simulink subsystem "PvtSubSys_VSM_LngHMI"  (R2020b)
settings: Solver=VariableStepAuto  StartTime=0.0  StopTime=10.0  RelTol=1e-3
undefined symbols (not defined in the file): ACC_STATE, HWA_STATE, P_VSM_HMI_Curve, P_VSM_HMI_CurveTime, P_VSM_LSMC_SampleTime, TJA_STATE
libraries: simulink x101
settings Model: Creator=GW00133806  LastModifiedBy=GW00201299

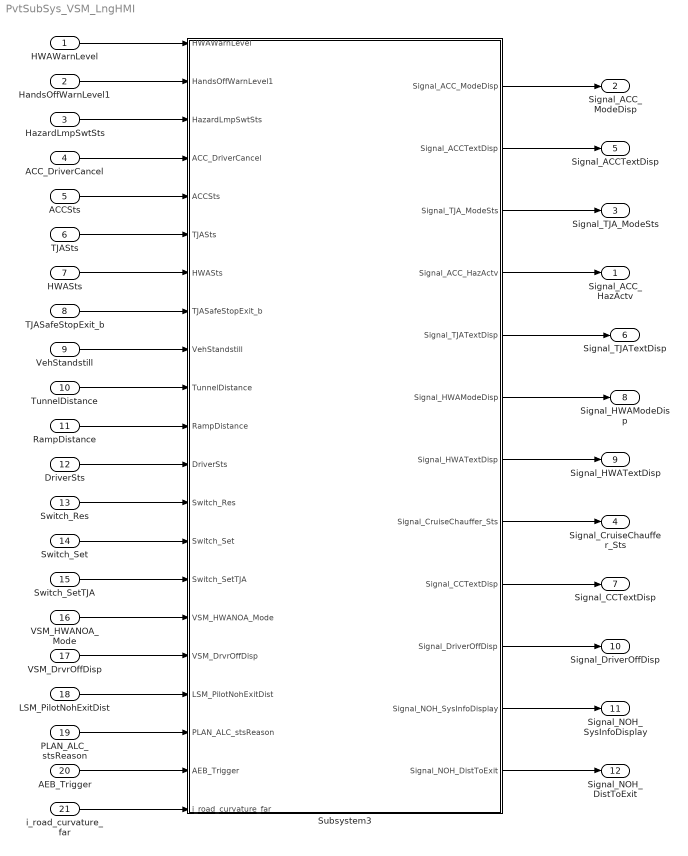
== system PvtSubSys_VSM_LngHMI ==
  HWAWarnLevel : Inport  OutDataTypeStr=uint8
  HandsOffWarnLevel1 : Inport  Port=2  OutDataTypeStr=uint8
  HazardLmpSwtSts : Inport  Port=3  OutDataTypeStr=boolean
  ACC_DriverCancel : Inport  Port=4  OutDataTypeStr=boolean
  ACCSts : Inport  Port=5  OutDataTypeStr=Enum: ACC_STATE
  TJASts : Inport  Port=6  OutDataTypeStr=Enum: TJA_STATE
  HWASts : Inport  Port=7  OutDataTypeStr=Enum: HWA_STATE
  TJASafeStopExit_b : Inport  Port=8  OutDataTypeStr=boolean
  VehStandstill : Inport  Port=9  OutDataTypeStr=uint8
  TunnelDistance : Inport  Port=10  OutDataTypeStr=uint16
  RampDistance : Inport  Port=11  OutDataTypeStr=uint16
  DriverSts : Inport  Port=12  OutDataTypeStr=uint8
  Switch_Res : Inport  Port=13  OutDataTypeStr=boolean
  Switch_Set : Inport  Port=14  OutDataTypeStr=boolean
  Switch_SetTJA : Inport  Port=15  OutDataTypeStr=boolean
  VSM_HWANOA_Mode : Inport  Port=16
  VSM_DrvrOffDisp : Inport  Port=17
  LSM_PilotNohExitDist : Inport  Port=18
  PLAN_ALC_stsReason : Inport  Port=19
  AEB_Trigger : Inport  Port=20
  i_road_curvature_far : Inport  Port=21
  Subsystem3 : Subsystem
  Signal_ACC_HazActv : Outport  OutDataTypeStr=uint8
  Signal_ACC_ModeDisp : Outport  Port=2  OutDataTypeStr=uint8
  Signal_TJA_ModeSts : Outport  Port=3  OutDataTypeStr=uint8
  Signal_CruiseChauffer_Sts : Outport  Port=4
  Signal_ACCTextDisp : Outport  Port=5  OutDataTypeStr=uint8
  Signal_TJATextDisp : Outport  Port=6  OutDataTypeStr=uint8
  Signal_CCTextDisp : Outport  Port=7
  Signal_HWAModeDisp : Outport  Port=8  OutDataTypeStr=uint8
  Signal_HWATextDisp : Outport  Port=9  OutDataTypeStr=uint8
  Signal_DriverOffDisp : Outport  Port=10
  Signal_NOH_SysInfoDisplay : Outport  Port=11
  Signal_NOH_DistToExit : Outport  Port=12
  wires:
  i_road_curvature_far/1 -> Subsystem3/21(i_road_curvature_far)
  AEB_Trigger/1 -> Subsystem3/20(AEB_Trigger)
  VSM_DrvrOffDisp/1 -> Subsystem3/17(VSM_DrvrOffDisp)
  VSM_HWANOA_Mode/1 -> Subsystem3/16(VSM_HWANOA_Mode)
  Switch_Set/1 -> Subsystem3/14(Switch_Set)
  TJASts/1 -> Subsystem3/6(TJASts)
  ACCSts/1 -> Subsystem3/5(ACCSts)
  HandsOffWarnLevel1/1 -> Subsystem3/2(HandsOffWarnLevel1)
  VehStandstill/1 -> Subsystem3/9(VehStandstill)
  ACC_DriverCancel/1 -> Subsystem3/4(ACC_DriverCancel)
  TJASafeStopExit_b/1 -> Subsystem3/8(TJASafeStopExit_b)
  TunnelDistance/1 -> Subsystem3/10(TunnelDistance)
  Switch_Res/1 -> Subsystem3/13(Switch_Res)
  RampDistance/1 -> Subsystem3/11(RampDistance)
  HWASts/1 -> Subsystem3/7(HWASts)
  HazardLmpSwtSts/1 -> Subsystem3/3(HazardLmpSwtSts)
  Subsystem3/7(Signal_HWATextDisp) -> Signal_HWATextDisp/1
  Subsystem3/1(Signal_ACC_ModeDisp) -> Signal_ACC_ModeDisp/1
  Subsystem3/8(Signal_CruiseChauffer_Sts) -> Signal_CruiseChauffer_Sts/1
  Subsystem3/9(Signal_CCTextDisp) -> Signal_CCTextDisp/1
  Switch_SetTJA/1 -> Subsystem3/15(Switch_SetTJA)
  Subsystem3/3(Signal_TJA_ModeSts) -> Signal_TJA_ModeSts/1
  Subsystem3/4(Signal_ACC_HazActv) -> Signal_ACC_HazActv/1
  HWAWarnLevel/1 -> Subsystem3/1(HWAWarnLevel)
  Subsystem3/2(Signal_ACCTextDisp) -> Signal_ACCTextDisp/1
  DriverSts/1 -> Subsystem3/12(DriverSts)
  Subsystem3/5(Signal_TJATextDisp) -> Signal_TJATextDisp/1
  Subsystem3/6(Signal_HWAModeDisp) -> Signal_HWAModeDisp/1
  Subsystem3/10(Signal_DriverOffDisp) -> Signal_DriverOffDisp/1
  LSM_PilotNohExitDist/1 -> Subsystem3/18(LSM_PilotNohExitDist)
  Subsystem3/11(Signal_NOH_SysInfoDisplay) -> Signal_NOH_SysInfoDisplay/1
  Subsystem3/12(Signal_NOH_DistToExit) -> Signal_NOH_DistToExit/1
  PLAN_ALC_stsReason/1 -> Subsystem3/19(PLAN_ALC_stsReason)

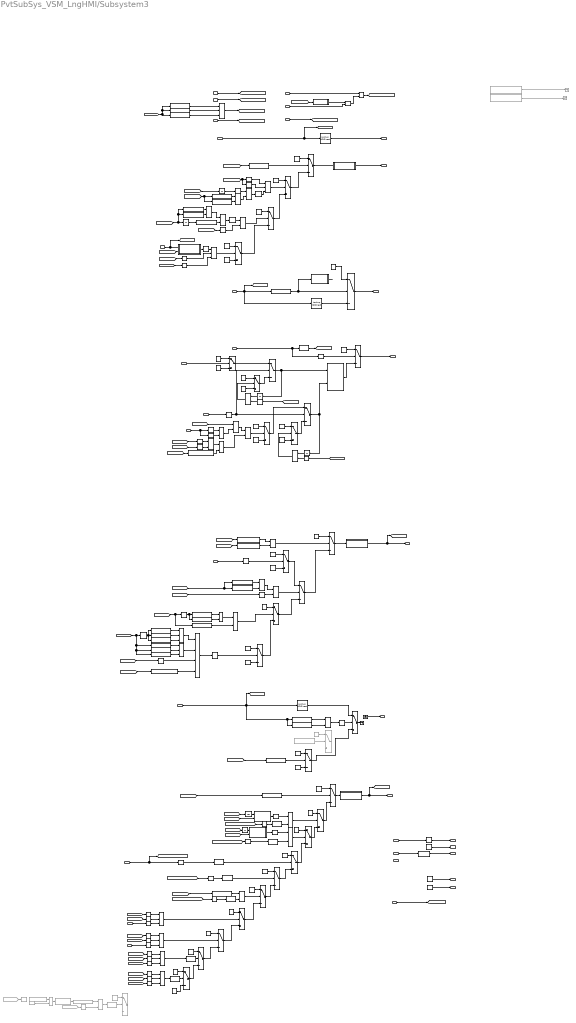
== system PvtSubSys_VSM_LngHMI/Subsystem3 ==
  note: 优先报ACC故障
  note: 0x0:No display
      | 0x1:Unable to activate TJA/ICA due to other limitation
      | 0x2:TJA/ICA active control is cancelled
      | 0x3:TJA/ICA   temporarily unavailable
      | 0x4:Current IGN Cycle Function Inhibit
      | 0x5：TJA Active
      | 0x6-0x7:Resvered
  note: 0x0:OFF
      | 0x1:Safstop
      | 0x2:Passive
      | 0x3:Ready
      | 0x4:Active
      | 0x5:Override
      | 0x6:Slow retreat
      | 0x7:Standstill
      | 0x8-0xE:Reserved
      | 0xF:Fault
  note: 0x0:No display
      | 0x1:Unable to activate HWA due to other limitation
      | 0x2:HWA active control is cancelled
      | 0x3:Turn off the turn light
      | 0x4:Active confirm
      | 0x5:Overtime for lane change
      | 0x6:lane change is cancelled
      | 0x7:HWA temporary unavailable
      | 0x8:Speed is too low to support lane change
      | 0x9:HWA need to restart the engine
      | 0xA:Take over request
      | 0xB: Please Keep Attention
      | 0xC:To cross the tunnel, please take over  in time
      | 0xD:Have a branch road ahead. Please take over in time
      | 0xE-0xF:Reserve
  note: 0x0:OFF mode
      | 0x1:Passive mode
      | 0x2:Active mode
      | 0x3:Ready
      | 0x4: Failure
      | 0x5:TJA_Wait状态灯闪闪烁，未确定此效果是否作出
  note: 0x00:No display
      | 0x01:Unable to activate ACC due to speed not achive
      | 0x02:ACC active control is cancelled
      | 0x03:Resvered
      | 0x04:ACC and PEBS temporary unavailable
      | 0x05:Unable to activate ACC due to other limitation(except speed not achive)
      | 0x06:ACC and PEBS error
      | 0x07:ACC temporary unavailable
      | 0x08:ACC Active
      | 0x09:Blindness
      | 0x0A-0x1F:Resvered
  note: 0x00:OFF Mode
      | 0x01:Passive Mode
      | 0x02:StandBy Mode
      | 0x03:Active-Control Mode
      | 0x04:Brake-Only Mode
      | 0x05:Override
      | 0X06:Reserved
      | 0X07:ACC and PEBS Failure mode
      | 0x08:ACC Failure mode
      | 0x09-0x1F:Reserved
  note: 2020.12.15
      | 1、新架构更新，初版
      |
      | 2020.12.29
      | 1、临时增加VSM_DrvrOffDisp信号输出到CCTextDisp上给HMI；
      | 2、修改HWA文字提醒输出3和5和8的逻辑；
      | 3、ACC仪表显示状态延迟2周期，以修改TJA激活时先报ACC激活的问题；
      | 4、TJA_Wait输出active到仪表；
      | 2021.1.5
      | 1、修改换道取消的发送逻辑，及其和换道成功的优先级顺序；
      | 2021.1.19
      | 把HWA的低速提醒限值改为PLAN的标定量；
      | 2021.1.27
      | ACC/TJA激活提醒策略添加；
      | 2021.1.30
      | TJA显示修改；
      | 2021.2.5
      | TJA显示修改；
      | ACC/TJA/HWA取消HMI逻辑修改
      | 2021.2.8
      | ACC/TJA故障显示优先级修改；
      | 2021.2.22
      | 增加NOH相关信号，增加ACCDrvrOffDisp信号；
      | 2021.3.5
      | VSM_HWA_ModeDisp删除override状态
      | 2021.3.12
      | TJA在ACCStandwait时不报退出提醒；
  note: 架构需求车速过低过
      | 高不能换道仅报警一次
  HWAWarnLevel : Inport  OutDataTypeStr=uint8
  HandsOffWarnLevel1 : Inport  Port=2  OutDataTypeStr=uint8
  HazardLmpSwtSts : Inport  Port=3  OutDataTypeStr=boolean
  ACC_DriverCancel : Inport  Port=4  OutDataTypeStr=boolean
  ACCSts : Inport  Port=5  OutDataTypeStr=Enum: ACC_STATE
  TJASts : Inport  Port=6  OutDataTypeStr=Enum: TJA_STATE
  HWASts : Inport  Port=7  OutDataTypeStr=Enum: HWA_STATE
  TJASafeStopExit_b : Inport  Port=8  OutDataTypeStr=boolean
  VehStandstill : Inport  Port=9  OutDataTypeStr=uint8
  TunnelDistance : Inport  Port=10  OutDataTypeStr=uint16
  RampDistance : Inport  Port=11  OutDataTypeStr=uint16
  DriverSts : Inport  Port=12  OutDataTypeStr=uint8
  Switch_Res : Inport  Port=13  OutDataTypeStr=boolean
  Switch_Set : Inport  Port=14  OutDataTypeStr=boolean
  Switch_SetTJA : Inport  Port=15  OutDataTypeStr=boolean
  VSM_HWANOA_Mode : Inport  Port=16
  VSM_DrvrOffDisp : Inport  Port=17
  LSM_PilotNohExitDist : Inport  Port=18
  PLAN_ALC_stsReason : Inport  Port=19
  AEB_Trigger : Inport  Port=20
  i_road_curvature_far : Inport  Port=21
  3-1跳变 : Stateflow chart  TreatAsAtomicUnit=on
  AND : Logic  AllPortsSameDT=off  OutDataTypeStr=boolean
  Abs : Abs  Commented=on
  Chart2 : Stateflow chart  TreatAsAtomicUnit=on
  Chart3 : Stateflow chart  TreatAsAtomicUnit=on
  Compare To Constant1 : simulink/Logic and Bit Operations/Compare To Constant  relop===  const=ACC_STATE.ACC_Failure  OutDataTypeStr=boolean
  Compare To Constant{2,10,12,19,22,40..41,44,47..48,51} (11 alike) : simulink/Logic and Bit Operations/Compare To Constant  relop===  const=1  OutDataTypeStr=boolean
  Compare To Constant104 : simulink/Logic and Bit Operations/Compare To Constant  relop===  const=7  OutDataTypeStr=boolean
  Compare To Constant{27,33,105..106} (4 alike) : simulink/Logic and Bit Operations/Compare To Constant  relop===  const=0  OutDataTypeStr=boolean
  Compare To Constant11 : simulink/Logic and Bit Operations/Compare To Constant  relop===  const=3  OutDataTypeStr=boolean
  Compare To Constant114 : simulink/Logic and Bit Operations/Compare To Constant  Commented=on  relop=>=  const=P_VSM_HMI_Curve  OutDataTypeStr=boolean
  Compare To Constant115 : simulink/Logic and Bit Operations/Compare To Constant  Commented=on  relop=<  const=1  OutDataTypeStr=boolean
  Compare To Constant116 : simulink/Logic and Bit Operations/Compare To Constant  Commented=on  relop=>  const=P_VSM_HMI_CurveTime  OutDataTypeStr=boolean
  Compare To Constant13 : simulink/Logic and Bit Operations/Compare To Constant  Commented=on  relop===  const=1  OutDataTypeStr=boolean
  Compare To Constant14 : simulink/Logic and Bit Operations/Compare To Constant  relop===  const=HWA_STATE.HWA_CCAct  OutDataTypeStr=boolean
  Compare To Constant15 : simulink/Logic and Bit Operations/Compare To Constant  relop===  const=HWA_STATE.HWA_Pause  OutDataTypeStr=boolean
  Compare To Constant16 : simulink/Logic and Bit Operations/Compare To Constant  Commented=on  relop===  const=ACC_STATE.ACC_Override  OutDataTypeStr=boolean
  Compare To Constant17 : simulink/Logic and Bit Operations/Compare To Constant  relop===  const=ACC_STATE.ACC_StandWait  OutDataTypeStr=boolean
  Compare To Constant18 : simulink/Logic and Bit Operations/Compare To Constant  relop=~=  const=ACC_STATE.ACC_StandWait  OutDataTypeStr=boolean
  Compare To Constant20 : simulink/Logic and Bit Operations/Compare To Constant  relop===  const=TJA_STATE.TJA_Idle  OutDataTypeStr=boolean
  Compare To Constant21 : simulink/Logic and Bit Operations/Compare To Constant  relop===  const=2  OutDataTypeStr=boolean
  Compare To Constant23 : simulink/Logic and Bit Operations/Compare To Constant  relop===  const=HWA_STATE.HWA_Error  OutDataTypeStr=boolean
  Compare To Constant24 : simulink/Logic and Bit Operations/Compare To Constant  relop===  const=TJA_STATE.TJA_Idle  OutDataTypeStr=boolean
  Compare To Constant25 : simulink/Logic and Bit Operations/Compare To Constant  relop===  const=TJA_STATE.TJA_SafeStop  OutDataTypeStr=boolean
  Compare To Constant26 : simulink/Logic and Bit Operations/Compare To Constant  relop===  const=TJA_STATE.TJA_Active  OutDataTypeStr=boolean
  Compare To Constant28 : simulink/Logic and Bit Operations/Compare To Constant  relop===  const=TJA_STATE.TJA_Wait  OutDataTypeStr=boolean
  Compare To Constant29 : simulink/Logic and Bit Operations/Compare To Constant  relop===  const=3  OutDataTypeStr=boolean
  Compare To Constant3 : simulink/Logic and Bit Operations/Compare To Constant  relop===  const=ACC_STATE.ACC_Reject  OutDataTypeStr=boolean
  Compare To Constant30 : simulink/Logic and Bit Operations/Compare To Constant  relop===  const=HWA_STATE.HWA_CCAct  OutDataTypeStr=boolean
  Compare To Constant31 : simulink/Logic and Bit Operations/Compare To Constant  relop===  const=TJA_STATE.TJA_Active  OutDataTypeStr=boolean
  Compare To Constant32 : simulink/Logic and Bit Operations/Compare To Constant  relop===  const=TJA_STATE.TJA_Wait  OutDataTypeStr=boolean
  Compare To Constant34 : simulink/Logic and Bit Operations/Compare To Constant  relop===  const=4  OutDataTypeStr=boolean
  Compare To Constant35 : simulink/Logic and Bit Operations/Compare To Constant  relop=~=  const=1  OutDataTypeStr=boolean
  Compare To Constant36 : simulink/Logic and Bit Operations/Compare To Constant  relop=~=  const=4  OutDataTypeStr=boolean
  Compare To Constant37 : simulink/Logic and Bit Operations/Compare To Constant  relop===  const=TJA_STATE.TJA_Ready  OutDataTypeStr=boolean
  Compare To Constant38 : simulink/Logic and Bit Operations/Compare To Constant  relop=~=  const=2  OutDataTypeStr=boolean
  Compare To Constant{39,43,46,49} (4 alike) : simulink/Logic and Bit Operations/Compare To Constant  relop=~=  const=0  OutDataTypeStr=boolean
  Compare To Constant4 : simulink/Logic and Bit Operations/Compare To Constant  relop===  const=ACC_STATE.ACC_Standby  OutDataTypeStr=boolean
  Compare To Constant42 : simulink/Logic and Bit Operations/Compare To Constant  relop=<=  const=300  OutDataTypeStr=boolean
  Compare To Constant45 : simulink/Logic and Bit Operations/Compare To Constant  relop=<=  const=300  OutDataTypeStr=boolean
  Compare To Constant5 : simulink/Logic and Bit Operations/Compare To Constant  relop===  const=2  OutDataTypeStr=boolean
  Compare To Constant50 : simulink/Logic and Bit Operations/Compare To Constant  relop=~=  const=1  OutDataTypeStr=boolean
  Compare To Constant52 : simulink/Logic and Bit Operations/Compare To Constant  relop===  const=TJA_STATE.TJA_SafeStop  OutDataTypeStr=boolean
  Compare To Constant53 : simulink/Logic and Bit Operations/Compare To Constant  relop=~=  const=2  OutDataTypeStr=boolean
  Compare To Constant54 : simulink/Logic and Bit Operations/Compare To Constant  relop===  const=TJA_STATE.TJA_SafeStop  OutDataTypeStr=boolean
  Compare To Constant55 : simulink/Logic and Bit Operations/Compare To Constant  relop===  const=TJA_STATE.TJA_SlowRetreat  OutDataTypeStr=boolean
  Compare To Constant56 : simulink/Logic and Bit Operations/Compare To Constant  relop=~=  const=ACC_STATE.ACC_Failure  OutDataTypeStr=boolean
  Compare To Constant58 : simulink/Logic and Bit Operations/Compare To Constant  relop=~=  const=5  OutDataTypeStr=boolean
  Compare To Constant59 : simulink/Logic and Bit Operations/Compare To Constant  relop===  const=ACC_STATE.ACC_Standby  OutDataTypeStr=boolean
  Compare To Constant6 : simulink/Logic and Bit Operations/Compare To Constant  relop===  const=3  OutDataTypeStr=boolean
  Compare To Constant60 : simulink/Logic and Bit Operations/Compare To Constant  relop===  const=ACC_STATE.ACC_ActiveControl  OutDataTypeStr=boolean
  Compare To Constant61 : simulink/Logic and Bit Operations/Compare To Constant  relop===  const=ACC_STATE.ACC_StandActive  OutDataTypeStr=boolean
  Compare To Constant63 : simulink/Logic and Bit Operations/Compare To Constant  relop===  const=TJA_STATE.TJA_Active  OutDataTypeStr=boolean
  Compare To Constant64 : simulink/Logic and Bit Operations/Compare To Constant  relop===  const=TJA_STATE.TJA_Ready  OutDataTypeStr=boolean
  Compare To Constant65 : simulink/Logic and Bit Operations/Compare To Constant  relop===  const=TJA_STATE.TJA_Error  OutDataTypeStr=boolean
  Compare To Constant66 : simulink/Logic and Bit Operations/Compare To Constant  relop===  const=TJA_STATE.TJA_Wait  OutDataTypeStr=boolean
  Compare To Constant67 : simulink/Logic and Bit Operations/Compare To Constant  relop===  const=TJA_STATE.TJA_Error  OutDataTypeStr=boolean
  Compare To Constant7 : simulink/Logic and Bit Operations/Compare To Constant  relop===  const=4  OutDataTypeStr=boolean
  Compare To Constant8 : simulink/Logic and Bit Operations/Compare To Constant  relop===  const=TJA_STATE.TJA_SlowRetreat  OutDataTypeStr=boolean
  Constant{,4,6..7,15,23,31,35,37,39} (10 alike) : Constant  Value=0  OutDataTypeStr=uint8
  Constant1 : Constant  Value=7  OutDataTypeStr=uint8
  Constant10 : Constant  Value=4  OutDataTypeStr=uint8
  Constant11 : Constant  Value=3  OutDataTypeStr=uint8
  Constant12 : Constant  Value=4  OutDataTypeStr=uint8
  Constant13 : Constant  OutDataTypeStr=uint8
  Constant{3,5,14,29} (4 alike) : Constant  Value=2  OutDataTypeStr=uint8
  Constant16 : Constant  Value=7  OutDataTypeStr=uint8
  Constant17 : Constant  Commented=on  Value=301  OutDataTypeStr=uint16
  Constant18 : Constant  Commented=on  Value=38252005  OutDataTypeStr=uint32
  Constant19 : Constant  Value=3  OutDataTypeStr=uint8
  Constant{2,21,32..33} (4 alike) : Constant  Value=5  OutDataTypeStr=uint8
  Constant22 : Constant  Value=8  OutDataTypeStr=uint8
  Constant24 : Constant  Value=12  OutDataTypeStr=uint8
  Constant25 : Constant  Value=13  OutDataTypeStr=uint8
  Constant26 : Constant  Value=10  OutDataTypeStr=uint8
  Constant27 : Constant  Value=11  OutDataTypeStr=uint8
  Constant28 : Constant  Value=8  OutDataTypeStr=uint8
  Constant30 : Constant  Value=6  OutDataTypeStr=uint8
  Constant34 : Constant  OutDataTypeStr=uint8
  Constant36 : Constant  Value=0  OutDataTypeStr=uint16
  Constant38 : Constant  OutDataTypeStr=uint8
  Constant54 : Constant  Value=15  OutDataTypeStr=uint8
  Constant56 : Constant  Commented=on  Value=14  OutDataTypeStr=uint8
  Constant8 : Constant  Commented=on  Value=5  OutDataTypeStr=uint8
  Constant9 : Constant  Value=7  OutDataTypeStr=uint8
  Data Type Conversion : DataTypeConversion
  Delay : Delay
  Delay1 : Delay  DelayLength=1  InitialCondition=TJA_STATE.TJA_Off
  Delay2 : Delay
  Delay3 : Delay  DelayLength=1  InitialCondition=TJA_STATE.TJA_Off
  Delay5 : Delay  DelayLength=3
  Delay6 : Delay  DelayLength=1  InitialCondition=0
  Detect Increase{,1..5,7,19} (8 alike) : simulink/Logic and Bit Operations/Detect Increase  vinit=0.0  OutDataTypeStr=boolean
  Detect Increase20 : simulink/Logic and Bit Operations/Detect Increase  Commented=on  vinit=0.0  OutDataTypeStr=boolean
  Direct Lookup Table (n-D)1 : LookupNDDirect  NumberOfTableDimensions=1  Table=[0 1 2 3 4 5 2 8 0 3]  TableDataTypeStr=uint8
  Direct Lookup Table (n-D)2 : LookupNDDirect  NumberOfTableDimensions=1  Table=[0 1 3 2 0 0 1 4 0 2 2]  TableDataTypeStr=uint8
  Direct Lookup Table (n-D)3 : LookupNDDirect  NumberOfTableDimensions=1  Table=[0 2 3 4 4 4 4 15 5 1 6]  TableDataTypeStr=uint8
  DriverSts_1 : InportShadow  Port=12  OutDataTypeStr=uint8
  Enlong3s : Subsystem
  Enlong3s1 : Subsystem
  Enlong3s2 : Subsystem
  From29 : From  Commented=on  GotoTag=HWAActive
  From81 : From  Commented=on  GotoTag=i_road_curvature_far
  Ground : Ground
  Logical Operator{,2,5..7,11,22,33,38} (9 alike) : Logic  Operator=OR  AllPortsSameDT=off  OutDataTypeStr=boolean
  Logical Operator{1,4,8..9,13..15,23,29,35..36,58..59} (13 alike) : Logic  AllPortsSameDT=off  OutDataTypeStr=boolean
  Logical Operator10 : Logic  Operator=NOT  Inputs=1  AllPortsSameDT=off  OutDataTypeStr=boolean
  Logical Operator12 : Logic  Operator=NOT  Inputs=1  AllPortsSameDT=off  OutDataTypeStr=boolean
  Logical Operator16 : Logic  Inputs=4  AllPortsSameDT=off  OutDataTypeStr=boolean
  Logical Operator17 : Logic  Operator=OR  Inputs=3  AllPortsSameDT=off  OutDataTypeStr=boolean
  Logical Operator18 : Logic  Operator=NOT  Inputs=1  AllPortsSameDT=off  OutDataTypeStr=boolean
  Logical Operator19 : Logic  Commented=on  AllPortsSameDT=off  OutDataTypeStr=boolean
  Logical Operator{25,27..28,30..32} (6 alike) : Logic  Inputs=3  AllPortsSameDT=off  OutDataTypeStr=boolean
  Logical Operator26 : Logic  Operator=OR  Inputs=3  AllPortsSameDT=off  OutDataTypeStr=boolean
  Logical Operator3 : Logic  Operator=OR  Inputs=3  AllPortsSameDT=off  OutDataTypeStr=boolean
  Logical Operator61 : Logic  Commented=on  AllPortsSameDT=off  OutDataTypeStr=boolean
  MATLAB Function : MATLAB Function  TreatAsAtomicUnit=on
  Subsystem : Subsystem
  Subsystem2 : Subsystem
  Subsystem9 : Subsystem  Commented=on  mask{Ts=P_VSM_LSMC_SampleTime, Max=10}
      mask prompts: Ts "Sample Time:"; Max "Max Limit:"
      mask Display:
      | Ts=get_param(gcb,'Ts');
      | Max=get_param(gcb,'Max');
      | disp(['Ts:' Ts '\n' 'Max:' Max ]);
  Switch{1..5,7,9..15,17,19..30,45} (27 alike) : Switch  Criteria=u2 ~= 0
  Switch16 : Switch  Criteria=u2 ~= 0  OutDataTypeStr=uint8
  Switch46 : Switch  Commented=on  Criteria=u2 ~= 0
  Switch6 : Switch  Criteria=u2 ~= 0  OutDataTypeStr=uint8
  Switch8 : Switch  Commented=on  Criteria=u2 ~= 0
  Terminator : Terminator
  Terminator6 : Terminator  Commented=on
  Terminator7 : Terminator  Commented=on
  Unit Delay{1,3..4,9..10} (5 alike) : UnitDelay  SampleTime=-1  HasFrameUpgradeWarning=on
  Unit Delay2 : UnitDelay  InitialCondition=ACC_STATE.ACC_Off  SampleTime=-1  HasFrameUpgradeWarning=on
  Signal_ACC_ModeDisp : Outport  OutDataTypeStr=uint8
  Signal_ACCTextDisp : Outport  Port=2  OutDataTypeStr=uint8
  Signal_TJA_ModeSts : Outport  Port=3  OutDataTypeStr=uint8
  Signal_ACC_HazActv : Outport  Port=4  OutDataTypeStr=uint8
  Signal_TJATextDisp : Outport  Port=5  OutDataTypeStr=uint8
  Signal_HWAModeDisp : Outport  Port=6  OutDataTypeStr=uint8
  Signal_HWATextDisp : Outport  Port=7  OutDataTypeStr=uint8
  Signal_CruiseChauffer_Sts : Outport  Port=8
  Signal_CCTextDisp : Outport  Port=9
  Signal_DriverOffDisp : Outport  Port=10
  Signal_NOH_SysInfoDisplay : Outport  Port=11
  Signal_NOH_DistToExit : Outport  Port=12
  wires:
  Constant18/1 -> Terminator6/1  "VSM_HMI_SubModel_VERSION"
  Constant17/1 -> Terminator7/1  "VSM_HMI_SubModel_Number"
  Logical Operator6/1 -> Logical Operator35/1
  Compare To Constant32/1 -> Logical Operator6/2
  Compare To Constant64/1 -> Logical Operator6/1
  Switch7/1 -> Terminator/1  "VSM_HWA_ModeDisp"
  Compare To Constant28/1 -> Logical Operator26/2
  Constant33/1 -> Switch29/1
  Detect Increase1/1 -> Switch24/2
  Detect Increase3/1 -> AND/2
  Compare To Constant30/1 -> AND/1
  [HWASts] -> Compare To Constant30/1
  Compare To Constant5/1 -> Detect Increase1/1
  Constant36/1 -> Signal_NOH_DistToExit/1
  Constant35/1 -> Signal_NOH_SysInfoDisplay/1
  Constant/1 -> Signal_CCTextDisp/1
  Compare To Constant37/1 -> Logical Operator26/3
  Constant4/1 -> Switch3/3
  [HWAWarnLevel] -> Compare To Constant46/1
  Logical Operator28/1 -> Detect Increase4/1
  Constant3/1 -> Switch3/1
  [TJATextDisp] -> Compare To Constant35/1, Compare To Constant36/1
  Constant7/1 -> Switch5/1
  Switch25/1 -> Switch14/3
  Switch10/1 -> Enlong3s/1(In1)
  TJASts/1 -> Compare To Constant66/1, Direct Lookup Table (n-D)2/1, [TJASts]
  Detect Increase2/1 -> Switch17/2
  Logical Operator8/1 -> Logical Operator33/1
  Constant26/1 -> Switch22/1
  Unit Delay1/1 -> Compare To Constant2/1
  Compare To Constant11/1 -> Logical Operator8/2
  [HWAActive] -> Compare To Constant51/1
  [TJASts] -> Compare To Constant52/1
  Constant9/1 -> Switch9/1
  Switch_Set/1 -> Logical Operator/1
  Detect Increase/1 -> [Hazlmp_Drvopr]
  [RampDistance] -> Compare To Constant45/1
  [ACCSts] -> Subsystem/2(ACCSts)
  Logical Operator27/1 -> Switch3/2
  Logical Operator38/1 -> Logical Operator14/1
  Subsystem/1(Out1) -> Delay5/1
  Constant16/1 -> Switch14/1
  Constant31/1 -> Switch26/3
  Constant29/1 -> Switch26/1
  Compare To Constant2/1 -> Logical Operator1/1
  Enlong3s2/1(Out1) -> [HWATextDisp], Signal_HWATextDisp/1  "VSM_HWATextDisp"
  Switch_SetTJA/1 -> [Switch_SetTJA]
  Switch26/1 -> Switch6/3
  [HWAWarnLevel] -> Compare To Constant49/1
  Switch22/1 -> Switch19/3
  [HWAActive] -> Compare To Constant41/1
  [ACC_Opration] -> Unit Delay1/1
  Logical Operator12/1 -> Switch7/2
  Constant10/1 -> Switch9/3
  [Switch_SetTJA] -> Compare To Constant40/1
  [ACCSts] -> Compare To Constant17/1
  Switch20/1 -> Switch23/3
  Constant6/1 -> Switch4/3
  [HWAWarnLevel] -> Compare To Constant11/1
  [TunnelDistance] -> Compare To Constant42/1
  Compare To Constant14/1 -> Logical Operator11/1
  Logical Operator4/1 -> Logical Operator7/1
  Constant14/1 -> Switch13/1
  ACC_DriverCancel/1 -> Subsystem/1(ACC_DriverCancel), [ACC_DriverCancel]
  Compare To Constant46/1 -> Logical Operator31/1
  [HWAWarnLevel] -> Compare To Constant43/1
  Constant11/1 -> Switch10/1
  Compare To Constant41/1 -> Logical Operator28/2
  Compare To Constant38/1 -> Logical Operator27/2
  Compare To Constant39/1 -> Logical Operator28/1
  Compare To Constant48/1 -> Logical Operator31/2
  Logical Operator7/1 -> Switch4/2
  Compare To Constant43/1 -> Logical Operator30/1
  Ground/1 -> Signal_HWAModeDisp/1  "VSM_HWA_ModeDisp"
  Logical Operator31/1 -> Switch22/2
  [ACCSts] -> Compare To Constant1/1
  Compare To Constant50/1 -> Logical Operator32/3
  Logical Operator9/1 -> Switch26/2
  Logical Operator25/1 -> Switch2/2
  Constant27/1 -> Switch23/1
  Compare To Constant36/1 -> Logical Operator25/2
  Compare To Constant40/1 -> Logical Operator14/2
  [HWAActive] -> Compare To Constant44/1
  Switch6/1 -> Unit Delay4/1, MATLAB Function/2(SafestopActive)
  RampDistance/1 -> [RampDistance]
  Compare To Constant15/1 -> Logical Operator11/2
  Logical Operator16/1 -> Delay6/1
  Compare To Constant33/1 -> Switch6/2, Switch16/2
  Switch21/1 -> Switch20/3
  Switch19/1 -> Switch17/3
  Compare To Constant42/1 -> Logical Operator28/3
  Compare To Constant51/1 -> Logical Operator32/2
  Switch23/1 -> Switch22/3
  HandsOffWarnLevel1/1 -> Compare To Constant7/1, Compare To Constant6/1
  [PLAN_ALC_stsReason] -> Compare To Constant29/1
  Compare To Constant17/1 -> Switch9/2
  DriverSts/1 -> Compare To Constant47/1
  Unit Delay4/1 -> Logical Operator9/1
  Detect Increase5/1 -> Switch21/2
  Switch9/1 -> Switch7/3
  Constant25/1 -> Switch21/1
  Direct Lookup Table (n-D)1/1 -> Signal_ACC_ModeDisp/1  "VSM_ACC_ModeDisp"
  TunnelDistance/1 -> [TunnelDistance]
  Compare To Constant45/1 -> Logical Operator30/3
  Constant23/1 -> Switch21/3
  AND/1 -> Switch19/2
  HWAWarnLevel/1 -> [HWAWarnLevel]
  Constant30/1 -> Switch24/1
  Switch5/1 -> Signal_ACC_HazActv/1  "VSM_ACC_HazActv"
  Switch2/1 -> Switch1/3
  Logical Operator5/1 -> Logical Operator4/2
  [ACC_DriverCancel] -> Compare To Constant27/1
  Compare To Constant44/1 -> Logical Operator30/2
  [HWAActive] -> Compare To Constant48/1
  DriverSts_1/1 -> Compare To Constant50/1
  [HWAActive] -> Logical Operator4/1
  Compare To Constant7/1 -> Logical Operator5/2
  Switch_Res/1 -> Logical Operator29/2
  Compare To Constant24/1 -> Logical Operator26/1
  Constant12/1 -> Switch12/1
  Enlong3s1/1(Out1) -> Signal_ACCTextDisp/1  "VSM_ACCTextDisp"
  Constant2/1 -> Switch2/1
  Compare To Constant3/1 -> Logical Operator2/1
  Compare To Constant4/1 -> Logical Operator2/2
  Compare To Constant49/1 -> Logical Operator32/1
  Compare To Constant35/1 -> Logical Operator25/1
  Delay/1 -> Logical Operator25/3
  [TJATextDisp] -> Compare To Constant38/1
  Compare To Constant27/1 -> Logical Operator16/3
  Logical Operator30/1 -> Detect Increase5/1
  Compare To Constant1/1 -> Switch1/2
  [HWAActive] -> Compare To Constant10/1
  [ACCSts] -> Subsystem2/1(In1)
  Constant8/1 -> Switch8/1
  Logical Operator1/1 -> Delay/1
  Constant5/1 -> Switch4/1
  Compare To Constant12/1 -> Switch5/2
  Constant1/1 -> Switch1/1
  [TJASts] -> Delay1/1, Compare To Constant37/1, Compare To Constant28/1, Compare To Constant24/1
  Compare To Constant6/1 -> Logical Operator5/1
  [Hazlmp_Drvopr] -> Logical Operator10/1
  Logical Operator29/1 -> Logical Operator/2
  Logical Operator10/1 -> Logical Operator9/2
  HWASts/1 -> Direct Lookup Table (n-D)3/1, [HWASts], Compare To Constant14/1, Compare To Constant15/1
  [ACCSts] -> Compare To Constant4/1, Compare To Constant3/1
  Compare To Constant47/1 -> Logical Operator31/3
  Compare To Constant52/1 -> Logical Operator33/2
  Compare To Constant16/1 -> Switch8/2
  Logical Operator32/1 -> Switch23/2
  TJASafeStopExit_b/1 -> Compare To Constant22/1
  Constant13/1 -> Switch12/3
  Logical Operator2/1 -> Logical Operator1/2
  Switch4/1 -> Switch6/1
  Logical Operator33/1 -> Logical Operator7/2
  [HWASts] -> Compare To Constant23/1
  Switch1/1 -> Enlong3s1/1(In1)
  Compare To Constant26/1 -> Logical Operator17/2
  Switch14/1 -> Enlong3s2/1(In1)
  [HWAWarnLevel] -> Compare To Constant39/1
  Enlong3s/1(Out1) -> [TJATextDisp], Signal_TJATextDisp/1  "VSM_TJATextDisp"
  Compare To Constant10/1 -> Logical Operator8/1
  Switch29/1 -> Signal_TJA_ModeSts/1  "VSM_TJA_ModeDisp"
  Constant24/1 -> Switch20/1
  Compare To Constant19/1 -> Detect Increase2/1
  Logical Operator14/1 -> Switch11/2
  Logical Operator11/1 -> Logical Operator12/1
  Constant21/1 -> Switch19/1
  [TJASts] -> Compare To Constant67/1, Compare To Constant20/1
  Detect Increase4/1 -> Switch20/2
  Compare To Constant22/1 -> Switch12/2
  Compare To Constant25/1 -> Logical Operator17/3
  Compare To Constant23/1 -> Switch14/2
  Logical Operator/1 -> [ACC_Opration]
  Logical Operator26/1 -> Logical Operator16/2
  Constant19/1 -> Switch17/1
  Constant15/1 -> Switch13/3
  Switch11/1 -> Switch10/3
  Subsystem2/1(Out1) -> Logical Operator29/1
  Switch12/1 -> Switch11/1
  Logical Operator17/1 -> Logical Operator16/1
  VSM_HWANOA_Mode/1 -> Compare To Constant21/1
  Compare To Constant21/1 -> Signal_CruiseChauffer_Sts/1
  VSM_DrvrOffDisp/1 -> Data Type Conversion/1
  Data Type Conversion/1 -> Signal_DriverOffDisp/1
  PLAN_ALC_stsReason/1 -> [PLAN_ALC_stsReason], Compare To Constant5/1
  Switch17/1 -> Switch24/3
  Switch27/1 -> Switch2/3
  Switch3/1 -> Switch27/3
  Constant28/1 -> Switch27/1
  Compare To Constant59/1 -> Logical Operator15/2
  Logical Operator22/1 -> Logical Operator15/1
  [ACCSts] -> Compare To Constant61/1, Compare To Constant60/1, Unit Delay2/1
  Compare To Constant61/1 -> Logical Operator22/2
  Compare To Constant60/1 -> Logical Operator22/1
  Unit Delay2/1 -> Compare To Constant59/1
  Logical Operator15/1 -> Delay2/1
  Logical Operator23/1 -> Switch27/2
  [TJATextDisp] -> Compare To Constant58/1
  Compare To Constant58/1 -> Logical Operator23/2
  Delay2/1 -> Logical Operator23/1
  Switch28/1 -> Switch11/3
  Switch13/1 -> Switch28/3
  Constant32/1 -> Switch28/1
  Compare To Constant63/1 -> Logical Operator35/2
  [TJASts] -> Compare To Constant63/1, Delay3/1
  Delay3/1 -> Compare To Constant64/1, Compare To Constant32/1
  Logical Operator35/1 -> Switch28/2
  Direct Lookup Table (n-D)2/1 -> Switch29/3
  Compare To Constant66/1 -> Switch29/2, 3-1跳变/1(Enable)
  Compare To Constant20/1 -> Logical Operator38/2
  Compare To Constant67/1 -> Logical Operator38/1
  3-1跳变/1(out) -> ?
  ACCSts/1 -> Direct Lookup Table (n-D)1/1, [ACCSts]
  Delay5/1 -> Logical Operator27/1
  Delay6/1 -> Switch13/2
  [HWATextDisp] -> Compare To Constant53/1
  Compare To Constant53/1 -> Logical Operator27/3
  Compare To Constant65/1 -> Logical Operator36/2
  [ACCSts] -> Compare To Constant56/1
  [TJASts] -> Compare To Constant65/1
  Compare To Constant56/1 -> Logical Operator36/1
  Logical Operator36/1 -> Switch10/2
  [PLAN_ALC_stsReason] -> Compare To Constant19/1
  Compare To Constant29/1 -> Detect Increase3/1
  Direct Lookup Table (n-D)3/1 -> Switch7/1
  Compare To Constant18/1 -> Logical Operator16/4
  [ACCSts] -> Compare To Constant18/1
  Compare To Constant54/1 -> Logical Operator3/2
  [TJASts] -> Compare To Constant31/1, Compare To Constant54/1, Compare To Constant55/1
  Compare To Constant31/1 -> Logical Operator3/1
  Logical Operator3/1 -> [HWAActive]
  Compare To Constant55/1 -> Logical Operator3/3
  Compare To Constant8/1 -> Logical Operator17/1
  Delay1/1 -> Compare To Constant25/1, Compare To Constant8/1, Compare To Constant26/1
  HazardLmpSwtSts/1 -> Compare To Constant12/1, Detect Increase/1
  MATLAB Function/1(y) -> Switch5/3
  Switch16/1 -> Unit Delay3/1, MATLAB Function/1(AEBactive)
  AEB_Trigger/1 -> Switch15/2
  Constant34/1 -> Switch15/1
  Constant37/1 -> Switch15/3
  Switch15/1 -> Switch16/1
  VehStandstill/1 -> Compare To Constant33/1
  Switch30/1 -> Switch16/3
  Constant38/1 -> Switch30/1
  Constant39/1 -> Switch30/3
  Logical Operator13/1 -> Switch30/2
  Logical Operator18/1 -> Logical Operator13/2
  [Hazlmp_Drvopr] -> Logical Operator18/1
  Unit Delay3/1 -> Logical Operator13/1
  i_road_curvature_far/1 -> [i_road_curvature_far]
  Detect Increase20/1 -> Switch46/2
  Subsystem9/1(Out1) -> Compare To Constant116/1
  Constant56/1 -> Switch46/1
  Compare To Constant114/1 -> Logical Operator61/1
  Logical Operator61/1 -> Subsystem9/1(In1)
  Compare To Constant115/1 -> Logical Operator61/2
  From81/1 -> Abs/1
  Compare To Constant116/1 -> Logical Operator19/1
  Logical Operator19/1 -> Detect Increase20/1
  From29/1 -> Compare To Constant13/1
  Compare To Constant13/1 -> Logical Operator19/2
  Compare To Constant105/1 -> Logical Operator58/1
  Compare To Constant106/1 -> Logical Operator59/1
  Unit Delay10/1 -> Chart3/1(HWATextDispK1)
  Compare To Constant34/1 -> Detect Increase7/1
  Chart3/1(y) -> Compare To Constant106/1
  Detect Increase19/1 -> Logical Operator59/2
  [HWATextDisp] -> Unit Delay9/1
  [PLAN_ALC_stsReason] -> Compare To Constant34/1
  Unit Delay9/1 -> Chart2/1(HWATextDispK1)
  Logical Operator59/1 -> Switch45/2
  Compare To Constant104/1 -> Detect Increase19/1
  [PLAN_ALC_stsReason] -> Compare To Constant104/1
  Logical Operator58/1 -> Switch25/2
  Constant54/1 -> Switch45/1
  Constant22/1 -> Switch25/1
  Detect Increase7/1 -> Logical Operator58/2
  [HWATextDisp] -> Unit Delay10/1
  Switch45/1 -> Switch25/3
  Chart2/1(y) -> Compare To Constant105/1
  Switch24/1 -> Switch45/3
  [TJASts] -> Chart2/2(TJASts)
  [TJASts] -> Chart3/2(TJASts)

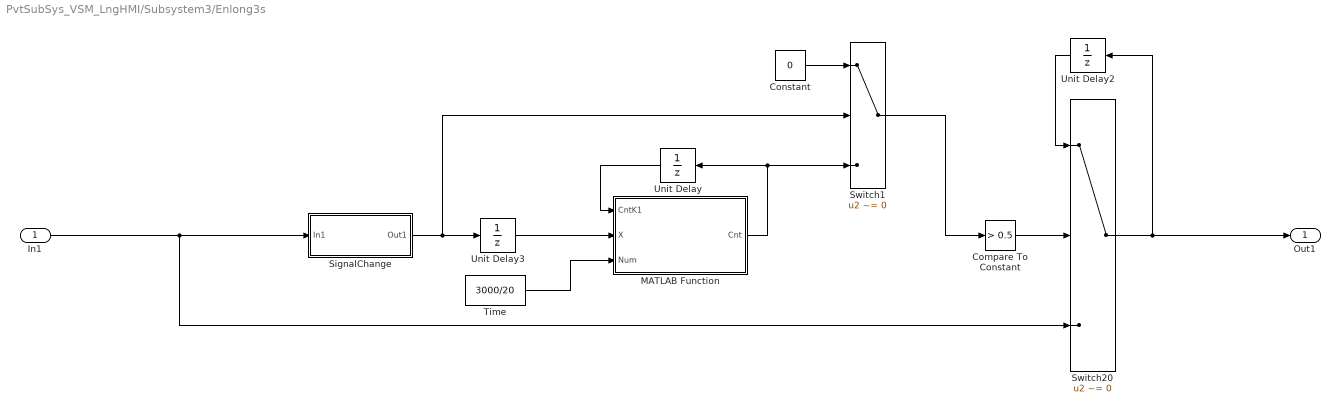
== system PvtSubSys_VSM_LngHMI/Subsystem3/Enlong3s ==
  In1 : Inport
  Compare To Constant : simulink/Logic and Bit Operations/Compare To Constant  relop=>  const=0.5  OutDataTypeStr=boolean
  Constant : Constant  Value=0  OutDataTypeStr=uint16
  MATLAB Function : MATLAB Function  TreatAsAtomicUnit=on
  SignalChange : Subsystem
  Switch1 : Switch  Criteria=u2 ~= 0
  Switch20 : Switch  Criteria=u2 ~= 0
  Time : Constant  Value=3000/20  OutDataTypeStr=uint16
  Unit Delay : UnitDelay  SampleTime=-1  HasFrameUpgradeWarning=on
  Unit Delay2 : UnitDelay  SampleTime=-1  HasFrameUpgradeWarning=on
  Unit Delay3 : UnitDelay  SampleTime=-1  HasFrameUpgradeWarning=on
  Out1 : Outport
  wires:
  In1/1 -> Switch20/3, SignalChange/1(In1)
  SignalChange/1(Out1) -> Switch1/2, Unit Delay3/1
  Unit Delay/1 -> MATLAB Function/1(CntK1)
  Constant/1 -> Switch1/1
  MATLAB Function/1(Cnt) -> Switch1/3, Unit Delay/1
  Switch1/1 -> Compare To Constant/1
  Compare To Constant/1 -> Switch20/2
  Unit Delay3/1 -> MATLAB Function/2(X)
  Unit Delay2/1 -> Switch20/1
  Switch20/1 -> Unit Delay2/1, Out1/1
  Time/1 -> MATLAB Function/3(Num)

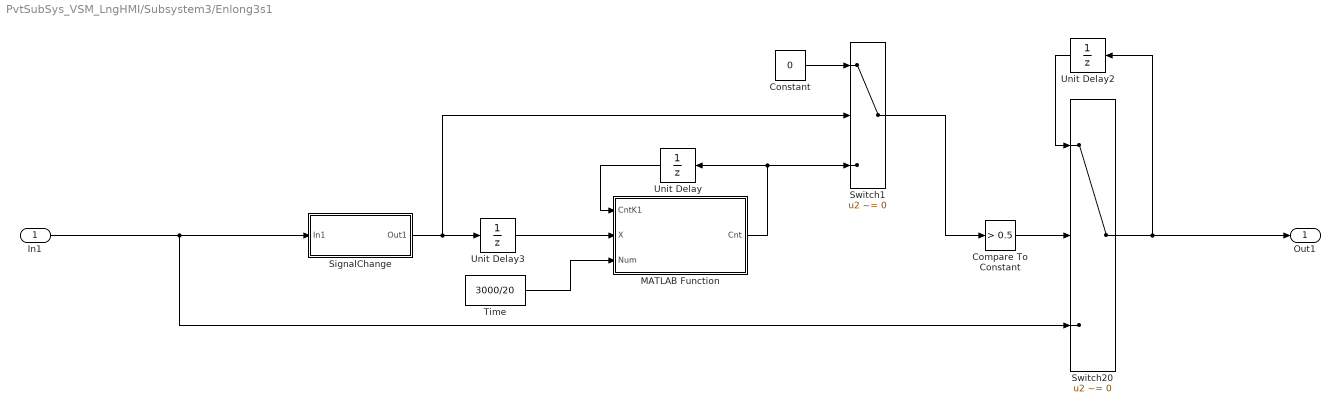
== system PvtSubSys_VSM_LngHMI/Subsystem3/Enlong3s1 ==
  In1 : Inport
  Compare To Constant : simulink/Logic and Bit Operations/Compare To Constant  relop=>  const=0.5  OutDataTypeStr=boolean
  Constant : Constant  Value=0  OutDataTypeStr=uint16
  MATLAB Function : MATLAB Function  TreatAsAtomicUnit=on
  SignalChange : Subsystem
  Switch1 : Switch  Criteria=u2 ~= 0
  Switch20 : Switch  Criteria=u2 ~= 0
  Time : Constant  Value=3000/20  OutDataTypeStr=uint16
  Unit Delay : UnitDelay  SampleTime=-1  HasFrameUpgradeWarning=on
  Unit Delay2 : UnitDelay  SampleTime=-1  HasFrameUpgradeWarning=on
  Unit Delay3 : UnitDelay  SampleTime=-1  HasFrameUpgradeWarning=on
  Out1 : Outport
  wires:
  Time/1 -> MATLAB Function/3(Num)
  Switch20/1 -> Out1/1, Unit Delay2/1
  Unit Delay2/1 -> Switch20/1
  Unit Delay3/1 -> MATLAB Function/2(X)
  Compare To Constant/1 -> Switch20/2
  Switch1/1 -> Compare To Constant/1
  MATLAB Function/1(Cnt) -> Unit Delay/1, Switch1/3
  Constant/1 -> Switch1/1
  Unit Delay/1 -> MATLAB Function/1(CntK1)
  SignalChange/1(Out1) -> Unit Delay3/1, Switch1/2
  In1/1 -> SignalChange/1(In1), Switch20/3

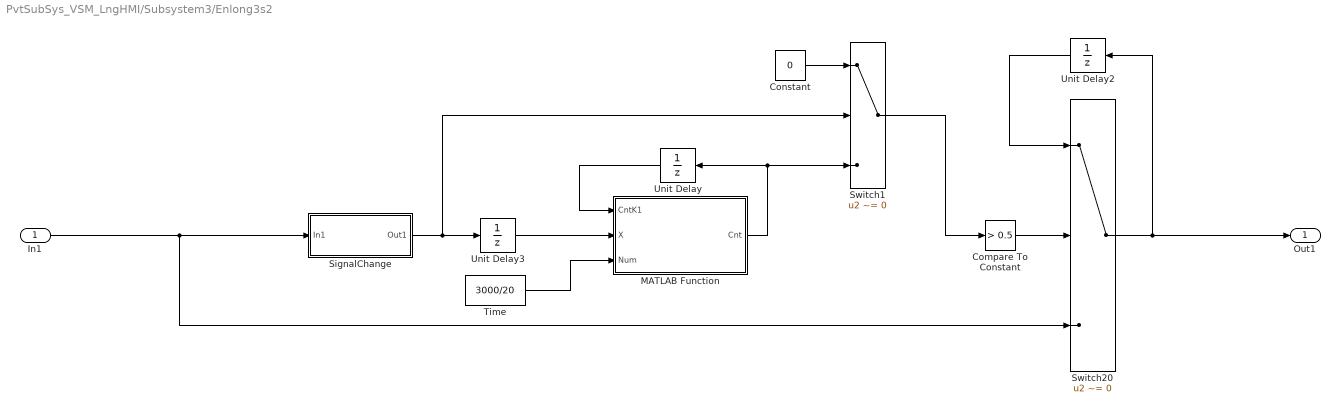
== system PvtSubSys_VSM_LngHMI/Subsystem3/Enlong3s2 ==
  In1 : Inport
  Compare To Constant : simulink/Logic and Bit Operations/Compare To Constant  relop=>  const=0.5  OutDataTypeStr=boolean
  Constant : Constant  Value=0  OutDataTypeStr=uint16
  MATLAB Function : MATLAB Function  TreatAsAtomicUnit=on
  SignalChange : Subsystem
  Switch1 : Switch  Criteria=u2 ~= 0
  Switch20 : Switch  Criteria=u2 ~= 0
  Time : Constant  Value=3000/20  OutDataTypeStr=uint16
  Unit Delay : UnitDelay  SampleTime=-1  HasFrameUpgradeWarning=on
  Unit Delay2 : UnitDelay  SampleTime=-1  HasFrameUpgradeWarning=on
  Unit Delay3 : UnitDelay  SampleTime=-1  HasFrameUpgradeWarning=on
  Out1 : Outport
  wires:
  In1/1 -> Switch20/3, SignalChange/1(In1)
  SignalChange/1(Out1) -> Switch1/2, Unit Delay3/1
  Unit Delay/1 -> MATLAB Function/1(CntK1)
  Constant/1 -> Switch1/1
  MATLAB Function/1(Cnt) -> Switch1/3, Unit Delay/1
  Switch1/1 -> Compare To Constant/1
  Compare To Constant/1 -> Switch20/2
  Unit Delay3/1 -> MATLAB Function/2(X)
  Unit Delay2/1 -> Switch20/1
  Switch20/1 -> Unit Delay2/1, Out1/1
  Time/1 -> MATLAB Function/3(Num)

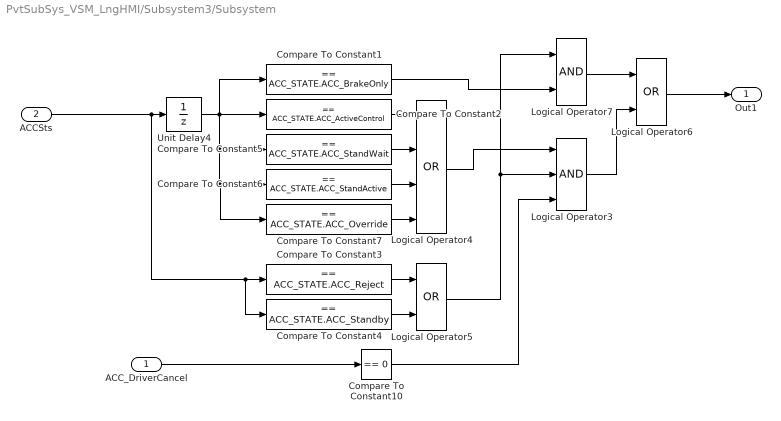
== system PvtSubSys_VSM_LngHMI/Subsystem3/Subsystem ==
  ACC_DriverCancel : Inport
  ACCSts : Inport  Port=2
  Compare To Constant1 : simulink/Logic and Bit Operations/Compare To Constant  relop===  const=ACC_STATE.ACC_BrakeOnly  OutDataTypeStr=boolean
  Compare To Constant10 : simulink/Logic and Bit Operations/Compare To Constant  relop===  const=0  OutDataTypeStr=boolean
  Compare To Constant2 : simulink/Logic and Bit Operations/Compare To Constant  relop===  const=ACC_STATE.ACC_ActiveControl  OutDataTypeStr=boolean
  Compare To Constant3 : simulink/Logic and Bit Operations/Compare To Constant  relop===  const=ACC_STATE.ACC_Reject  OutDataTypeStr=boolean
  Compare To Constant4 : simulink/Logic and Bit Operations/Compare To Constant  relop===  const=ACC_STATE.ACC_Standby  OutDataTypeStr=boolean
  Compare To Constant5 : simulink/Logic and Bit Operations/Compare To Constant  relop===  const=ACC_STATE.ACC_StandWait  OutDataTypeStr=boolean
  Compare To Constant6 : simulink/Logic and Bit Operations/Compare To Constant  relop===  const=ACC_STATE.ACC_StandActive  OutDataTypeStr=boolean
  Compare To Constant7 : simulink/Logic and Bit Operations/Compare To Constant  relop===  const=ACC_STATE.ACC_Override  OutDataTypeStr=boolean
  Logical Operator3 : Logic  Inputs=3  AllPortsSameDT=off  OutDataTypeStr=boolean
  Logical Operator4 : Logic  Operator=OR  Inputs=4  AllPortsSameDT=off  OutDataTypeStr=boolean
  Logical Operator5 : Logic  Operator=OR  AllPortsSameDT=off  OutDataTypeStr=boolean
  Logical Operator6 : Logic  Operator=OR  AllPortsSameDT=off  OutDataTypeStr=boolean
  Logical Operator7 : Logic  AllPortsSameDT=off  OutDataTypeStr=boolean
  Unit Delay4 : UnitDelay  InitialCondition=ACC_STATE.ACC_Off  SampleTime=-1  HasFrameUpgradeWarning=on
  Out1 : Outport
  wires:
  Compare To Constant7/1 -> Logical Operator4/4
  Compare To Constant6/1 -> Logical Operator4/3
  Compare To Constant5/1 -> Logical Operator4/2
  Compare To Constant1/1 -> Logical Operator7/2
  Compare To Constant2/1 -> Logical Operator4/1
  Compare To Constant3/1 -> Logical Operator5/1
  Compare To Constant4/1 -> Logical Operator5/2
  ACCSts/1 -> Unit Delay4/1, Compare To Constant4/1, Compare To Constant3/1
  Unit Delay4/1 -> Compare To Constant5/1, Compare To Constant6/1, Compare To Constant7/1, Compare To Constant2/1, Compare To Constant1/1
  Logical Operator7/1 -> Logical Operator6/1
  Compare To Constant10/1 -> Logical Operator3/3
  ACC_DriverCancel/1 -> Compare To Constant10/1
  Logical Operator3/1 -> Logical Operator6/2
  Logical Operator4/1 -> Logical Operator3/1
  Logical Operator6/1 -> Out1/1
  Logical Operator5/1 -> Logical Operator3/2, Logical Operator7/1

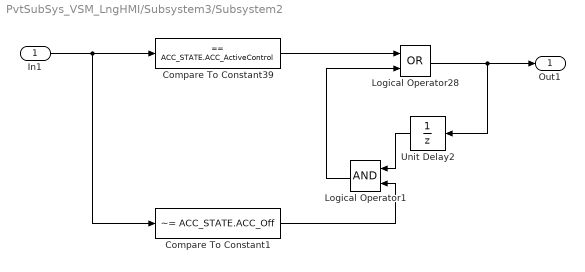
== system PvtSubSys_VSM_LngHMI/Subsystem3/Subsystem2 ==
  In1 : Inport
  Compare To Constant1 : simulink/Logic and Bit Operations/Compare To Constant  relop=~=  const=ACC_STATE.ACC_Off  OutDataTypeStr=boolean
  Compare To Constant39 : simulink/Logic and Bit Operations/Compare To Constant  relop===  const=ACC_STATE.ACC_ActiveControl  OutDataTypeStr=boolean
  Logical Operator1 : Logic  AllPortsSameDT=off  OutDataTypeStr=boolean
  Logical Operator28 : Logic  Operator=OR  AllPortsSameDT=off  OutDataTypeStr=boolean
  Unit Delay2 : UnitDelay  SampleTime=-1  HasFrameUpgradeWarning=on
  Out1 : Outport
  wires:
  Compare To Constant1/1 -> Logical Operator1/2
  Logical Operator1/1 -> Logical Operator28/2
  In1/1 -> Compare To Constant1/1, Compare To Constant39/1
  Unit Delay2/1 -> Logical Operator1/1
  Logical Operator28/1 -> Unit Delay2/1, Out1/1
  Compare To Constant39/1 -> Logical Operator28/1

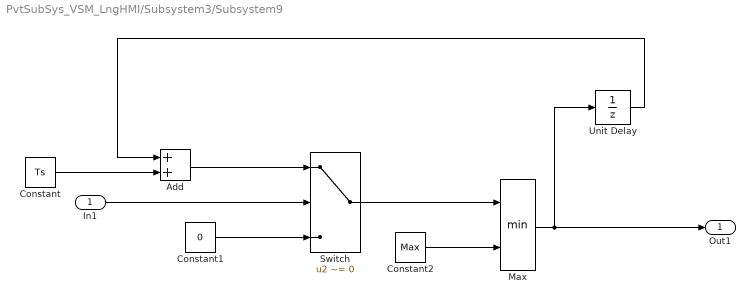
== system PvtSubSys_VSM_LngHMI/Subsystem3/Subsystem9 ==
  In1 : Inport
  Add : Sum
  Constant : Constant  Value=Ts
  Constant1 : Constant  Value=0
  Constant2 : Constant  Value=Max
  Max : MinMax  Inputs=2
  Switch : Switch  Criteria=u2 ~= 0
  Unit Delay : UnitDelay  SampleTime=-1  HasFrameUpgradeWarning=on
  Out1 : Outport
  wires:
  Unit Delay/1 -> Add/1
  In1/1 -> Switch/2
  Constant/1 -> Add/2
  Constant1/1 -> Switch/3
  Add/1 -> Switch/1
  Max/1 -> Unit Delay/1, Out1/1
  Constant2/1 -> Max/2
  Switch/1 -> Max/1

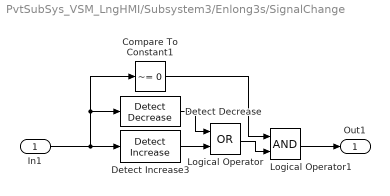
== system PvtSubSys_VSM_LngHMI/Subsystem3/Enlong3s/SignalChange ==
  In1 : Inport
  Compare To Constant1 : simulink/Logic and Bit Operations/Compare To Constant  relop=~=  const=0  OutDataTypeStr=boolean
  Detect Decrease : simulink/Logic and Bit Operations/Detect Decrease  vinit=0.0  OutDataTypeStr=boolean
  Detect Increase3 : simulink/Logic and Bit Operations/Detect Increase  vinit=0.0  OutDataTypeStr=boolean
  Logical Operator : Logic  Operator=OR  AllPortsSameDT=off  OutDataTypeStr=boolean
  Logical Operator1 : Logic  AllPortsSameDT=off  OutDataTypeStr=boolean
  Out1 : Outport
  wires:
  In1/1 -> Detect Increase3/1, Detect Decrease/1, Compare To Constant1/1
  Detect Increase3/1 -> Logical Operator/2
  Compare To Constant1/1 -> Logical Operator1/1
  Logical Operator1/1 -> Out1/1
  Logical Operator/1 -> Logical Operator1/2
  Detect Decrease/1 -> Logical Operator/1

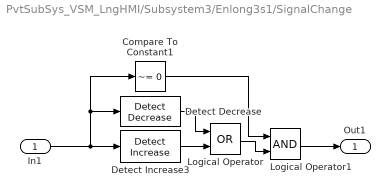
== system PvtSubSys_VSM_LngHMI/Subsystem3/Enlong3s1/SignalChange ==
  In1 : Inport
  Compare To Constant1 : simulink/Logic and Bit Operations/Compare To Constant  relop=~=  const=0  OutDataTypeStr=boolean
  Detect Decrease : simulink/Logic and Bit Operations/Detect Decrease  vinit=0.0  OutDataTypeStr=boolean
  Detect Increase3 : simulink/Logic and Bit Operations/Detect Increase  vinit=0.0  OutDataTypeStr=boolean
  Logical Operator : Logic  Operator=OR  AllPortsSameDT=off  OutDataTypeStr=boolean
  Logical Operator1 : Logic  AllPortsSameDT=off  OutDataTypeStr=boolean
  Out1 : Outport
  wires:
  Detect Decrease/1 -> Logical Operator/1
  Logical Operator/1 -> Logical Operator1/2
  Logical Operator1/1 -> Out1/1
  Compare To Constant1/1 -> Logical Operator1/1
  Detect Increase3/1 -> Logical Operator/2
  In1/1 -> Compare To Constant1/1, Detect Decrease/1, Detect Increase3/1

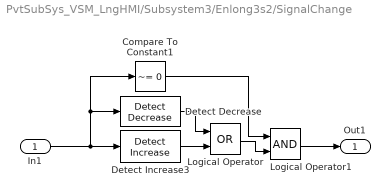
== system PvtSubSys_VSM_LngHMI/Subsystem3/Enlong3s2/SignalChange ==
  In1 : Inport
  Compare To Constant1 : simulink/Logic and Bit Operations/Compare To Constant  relop=~=  const=0  OutDataTypeStr=boolean
  Detect Decrease : simulink/Logic and Bit Operations/Detect Decrease  vinit=0.0  OutDataTypeStr=boolean
  Detect Increase3 : simulink/Logic and Bit Operations/Detect Increase  vinit=0.0  OutDataTypeStr=boolean
  Logical Operator : Logic  Operator=OR  AllPortsSameDT=off  OutDataTypeStr=boolean
  Logical Operator1 : Logic  AllPortsSameDT=off  OutDataTypeStr=boolean
  Out1 : Outport
  wires:
  In1/1 -> Detect Increase3/1, Detect Decrease/1, Compare To Constant1/1
  Detect Increase3/1 -> Logical Operator/2
  Compare To Constant1/1 -> Logical Operator1/1
  Logical Operator1/1 -> Out1/1
  Logical Operator/1 -> Logical Operator1/2
  Detect Decrease/1 -> Logical Operator/1

== stateflow chart PvtSubSys_VSM_LngHMI/Subsystem3/3-1跳变 ==
  state Initial
    out=uint8(1);
  state Ready
    en:
    out=uint8(3);
    cnt=0;
    du:
    cnt=min(100,cnt+1)
  state Passive
    en:
    out=uint8(1);
    cnt=0;
    du:
    cnt=min(100,cnt+1)
  (default) -> Initial
  Initial -> Ready : [Enable==true]
  Ready -> Initial [order 2] : [Enable==false]
  Passive -> Initial [order 2] : [[Enable==false]]
  Ready -> Passive [order 1] : [cnt>25]
  Passive -> Ready [order 1] : [cnt>25]
  data: out output uint8; Enable input boolean; cnt local

== matlab function PvtSubSys_VSM_LngHMI/Subsystem3/Enlong3s/MATLAB Function ==
  data: CntK1 input uint16; Cnt output uint16; X input; Num input
function Cnt= TextCount(CntK1,X,Num)

if X==true
    Cnt = Num;
else
     Cnt = max(CntK1-uint16(1),uint16(0));
end

== matlab function PvtSubSys_VSM_LngHMI/Subsystem3/Enlong3s1/MATLAB Function ==
  data: CntK1 input uint16; Cnt output uint16; X input; Num input
function Cnt= TextCount(CntK1,X,Num)

if X==true
    Cnt = Num;
else
     Cnt = max(CntK1-uint16(1),uint16(0));
end

== matlab function PvtSubSys_VSM_LngHMI/Subsystem3/Enlong3s2/MATLAB Function ==
  data: CntK1 input uint16; Cnt output uint16; X input; Num input
function Cnt= TextCount(CntK1,X,Num)

if X==true
    Cnt = Num;
else
     Cnt = max(CntK1-uint16(1),uint16(0));
end

== stateflow chart PvtSubSys_VSM_LngHMI/Subsystem3/Chart3 ==
  state NoActive
    en:
    y=0;
  state Active
    en:
    y=1;
  (default) -> NoActive
  NoActive -> Active : [HWATextDispK1==15 ]
  Active -> NoActive : [TJASts==TJA_STATE.TJA_Idle||TJASts==TJA_STATE.TJA_Off||TJASts==TJA_STATE.TJA_Ready]
  data: HWATextDispK1 input; y output; TJASts input

== matlab function PvtSubSys_VSM_LngHMI/Subsystem3/MATLAB Function ==
  data: AEBactive input; y output uint8; SafestopActive input
function y = fcn(AEBactive, SafestopActive)
y=uint8(0);
if AEBactive>uint8(0)
    y=AEBactive;
elseif SafestopActive>uint8(0)
    y=SafestopActive;
end

== stateflow chart PvtSubSys_VSM_LngHMI/Subsystem3/Chart2 ==
  state NoActive
    en:
    y=0;
  state Active
    en:
    y=1;
  (default) -> NoActive
  NoActive -> Active : [HWATextDispK1==8 ]
  Active -> NoActive : [TJASts==TJA_STATE.TJA_Idle||TJASts==TJA_STATE.TJA_Off||TJASts==TJA_STATE.TJA_Ready]
  data: HWATextDispK1 input; y output; TJASts input
